simulink model "Origem"  (R2017a)
settings: Solver=VariableStepAuto  StartTime=0.0  StopTime=100  RelTol=1e-3
values from neighbouring files (symbols this model uses):
  A0 = pi/2    (= 1.57079632679)    [main.m]
  omega = 2 * pi * Raio    (= 62.8318530718)    [main.m]
  ve0 = omega * Raio    (= 628.318530718)    [main.m]
  vn0 = 0    [main.m]
  xe0 = 0    [main.m]
  xn0 = Raio    (= 10)    [main.m]
libraries: simulink x1
settings Model: Creator=eduardo  LastModifiedBy=eduardo

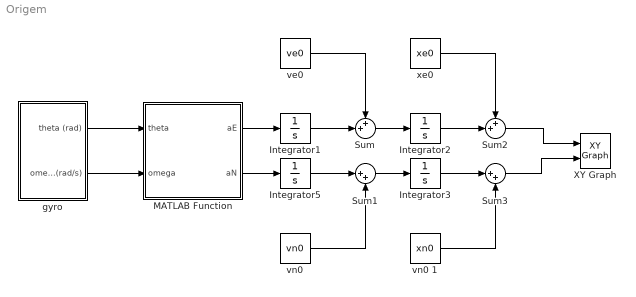
== system Origem ==
  Integrator{1..3,5} (4 alike) : Integrator
  MATLAB Function : MATLAB Function  TreatAsAtomicUnit=on
  Sum : Sum  Inputs=++|
  Sum1 : Sum  Inputs=|++
  Sum2 : Sum  Inputs=++|
  Sum3 : Sum  Inputs=|++
  XY Graph : simulink/Sinks/XY Graph  xmin=-15  xmax=15  ymin=-15  ymax=15  st=-1
  gyro : Subsystem
  ve0 : Constant  Value=ve0
  "vn0 " : Constant  Value=vn0
  vn0 1 : Constant  Value=xn0
  xe0 : Constant  Value=xe0
  wires:
  gyro/2(omega (rad/s)) -> MATLAB Function/2(omega)
  gyro/1(theta (rad)) -> MATLAB Function/1(theta)
  MATLAB Function/1(aE) -> Integrator1/1
  Integrator1/1 -> Sum/2
  ve0/1 -> Sum/1
  Integrator5/1 -> Sum1/1
  "vn0 "/1 -> Sum1/2
  xe0/1 -> Sum2/1
  Integrator2/1 -> Sum2/2
  vn0 1/1 -> Sum3/2
  Integrator3/1 -> Sum3/1
  MATLAB Function/2(aN) -> Integrator5/1
  Sum1/1 -> Integrator3/1
  Sum/1 -> Integrator2/1
  Sum2/1 -> XY Graph/1
  Sum3/1 -> XY Graph/2

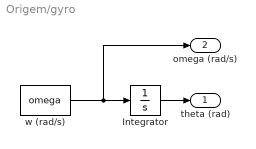
== system Origem/gyro ==
  Integrator : Integrator  InitialCondition=A0
  w (rad/s) : Constant  Value=omega
  theta (rad) : Outport
  omega (rad/s) : Outport  Port=2
  wires:
  w (rad/s)/1 -> omega (rad/s)/1, Integrator/1
  Integrator/1 -> theta (rad)/1

== matlab function Origem/MATLAB Function ==
  data: aE output; aN output; theta input; omega input
function [aE, aN]= fun(theta, omega)

R = 10;

ax = omega^2 * R;
ay = 0;

Ab = [ax ay]';
% Saída.
% ======
R_b2n = [ +cos(theta)   sin(theta);
          -sin(theta)   cos(theta)];
      
R = R_b2n * Ab;
aE = R(1);
aN = R(2);
